simulink library "INT_CoVM_SpdCoord"  (R2016b)
settings: Solver=VariableStepAuto  StartTime=0.0  StopTime=10.0  RelTol=1e-3
settings Model: Creator=Administrator  LastModifiedBy=Administrator

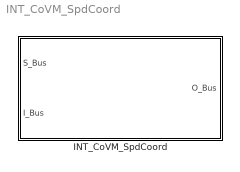
== system INT_CoVM_SpdCoord ==
  INT_CoVM_SpdCoord : Subsystem

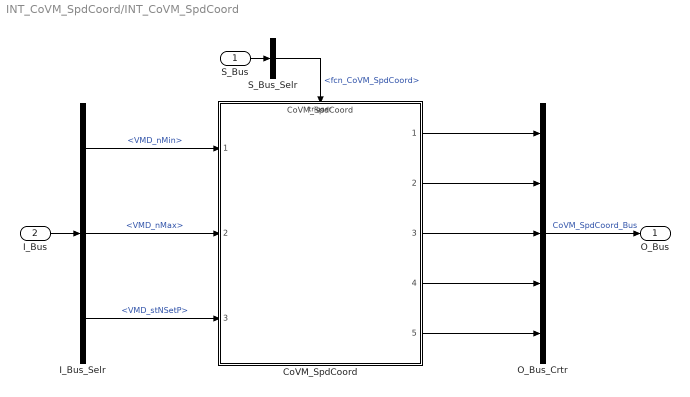
== system INT_CoVM_SpdCoord/INT_CoVM_SpdCoord ==
  S_Bus : Inport
  I_Bus : Inport  Port=2
  CoVM_SpdCoord : ModelReference  ModelNameDialog=CoVM_SpdCoord  SimulationMode=Normal  ModelReferenceVersion=1.5  TriggerPortName=function  TriggerPortTriggerType=function-call  TriggerPortStatesWhenEnabling=held
  I_Bus_Selr : BusSelector  OutputSignals=VMD_nMin,VMD_nMax,VMD_stNSetP
  O_Bus_Crtr : BusCreator  Inputs=5
  S_Bus_Selr : BusSelector  OutputSignals=fcn_CoVM_SpdCoord
  O_Bus : Outport
  wires:
  S_Bus_Selr/1 -> CoVM_SpdCoord/Trigger  "<fcn_CoVM_SpdCoord>"
  S_Bus/1 -> S_Bus_Selr/1
  I_Bus/1 -> I_Bus_Selr/1
  I_Bus_Selr/1 -> CoVM_SpdCoord/1  "<VMD_nMin>"
  I_Bus_Selr/2 -> CoVM_SpdCoord/2  "<VMD_nMax>"
  I_Bus_Selr/3 -> CoVM_SpdCoord/3  "<VMD_stNSetP>"
  O_Bus_Crtr/1 -> O_Bus/1  "CoVM_SpdCoord_Bus"
  CoVM_SpdCoord/1 -> O_Bus_Crtr/1
  CoVM_SpdCoord/2 -> O_Bus_Crtr/2
  CoVM_SpdCoord/3 -> O_Bus_Crtr/3
  CoVM_SpdCoord/4 -> O_Bus_Crtr/4
  CoVM_SpdCoord/5 -> O_Bus_Crtr/5
